simulink model "randomrotation_subsystem"  (R2023b)
settings: Solver=VariableStepAuto  StartTime=0.0  StopTime=30.0  RelTol=1e-3
settings Model: Creator=branko  LastModifiedBy=branko

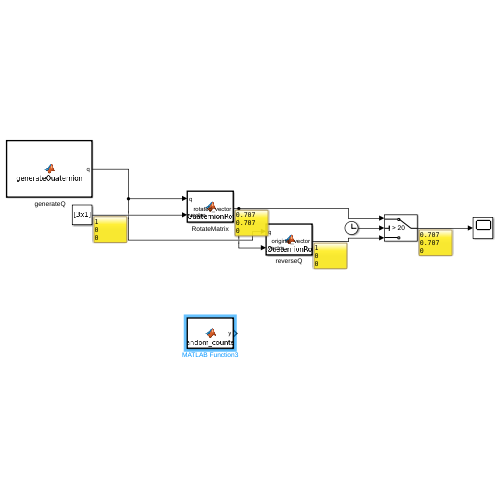
[thumbnail: Simulink's stored preview of the top-level diagram]
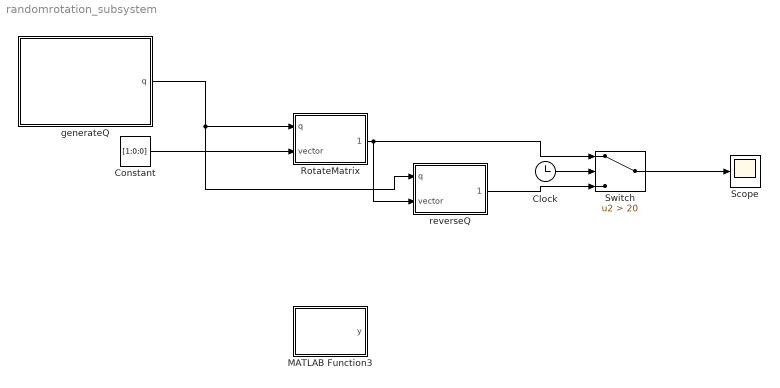
== system randomrotation_subsystem ==
  " generateQ" : MATLAB Function  TreatAsAtomicUnit=on
  Clock : Clock
  Constant : Constant  Value=[1;0;0]
  MATLAB Function3 : MATLAB Function  TreatAsAtomicUnit=on
  RotateMatrix : MATLAB Function  TreatAsAtomicUnit=on
  Scope : Scope
  Switch : Switch  Criteria=u2 > Threshold  Threshold=20  SaturateOnIntegerOverflow=off  InputSameDT=off
  reverseQ : MATLAB Function  TreatAsAtomicUnit=on
  wires:
  " generateQ"/1(q) -> reverseQ/1(q), RotateMatrix/1(q)
  Constant/1 -> RotateMatrix/2(vector)
  reverseQ/1(original_vector) -> Switch/3
  RotateMatrix/1(rotated_vector) -> Switch/1, reverseQ/2(vector)
  Clock/1 -> Switch/2
  Switch/1 -> Scope/1

== matlab function randomrotation_subsystem/ generateQ ==
  data: q output
function q = generateQuaternion()
    % Define the angle in radians (45 degrees)
    angle_radians = deg2rad(45);
    % Fixed axis (e.g., z-axis)
    axis = [0; 0; 1];
    % Calculate the quaternion
    q = [cos(angle_radians / 2); sin(angle_radians / 2) * axis];
end

== matlab function randomrotation_subsystem/reverseQ ==
  data: q input; original_vector output; vector input
function original_vector = revertQuaternionRotation(q, vector)
    % Extract quaternion components
    w = q(1);
    x = -q(2);
    y = -q(3);
    z = -q(4);
    % Inverse quaternion (conjugate for unit quaternion)
     % q_inv = [w; -x; -y; -z];
    % Apply inverse rotation
         % Quaternion rotation matrix
    R = [1 - 2*y^2 - 2*z^2, 2*x*y - 2*z*w, 2*x*z + 2*y*w;
         2*x*y + 2*z*w, 1 - 2*x^2 - 2*z^2, 2*y*z - 2*x*w;
         2*x*z - 2*y*w, 2*y*z + 2*x*w, 1 - 2*x^2 - 2*y^2];
    % Apply rotation
    original_vector = R * vector;
end

== matlab function randomrotation_subsystem/MATLAB Function3 ==
  data: y output
function y = random_counter()
    persistent counter;
    
    % Initialize counter if not already initialized
    if isempty(counter)
        counter = 0;
    end
    
    % Increment counter
    counter = counter + 1;
    
    % Check if counter has reached a random interval between 0 and 20
    if counter >= randi([10, 30])
        % Reset counter to 0
        counter = 0;
    end
    
    y = counter;
end

== matlab function randomrotation_subsystem/RotateMatrix ==
  data: q input; rotated_vector output; vector input
function rotated_vector = applyQuaternionRotation(q, vector)
    % Extract quaternion components
    w = q(1);
    x = q(2);
    y = q(3);
    z = q(4);
    % Quaternion rotation matrix
    R = [1 - 2*y^2 - 2*z^2, 2*x*y - 2*z*w, 2*x*z + 2*y*w;
         2*x*y + 2*z*w, 1 - 2*x^2 - 2*z^2, 2*y*z - 2*x*w;
         2*x*z - 2*y*w, 2*y*z + 2*x*w, 1 - 2*x^2 - 2*y^2];
    % Apply rotation
    rotated_vector = R * vector;
end
